simulink model "task3"  (R2024a)
settings: Solver=VariableStepAuto  StartTime=0.0  StopTime=10.0  MaxStep=0.1  RelTol=1e-3
undefined symbols (not defined in the file): A, B, C, D, K, L, x0, x0_hat
settings Model: Creator=sizgr  LastModifiedBy=sizgr

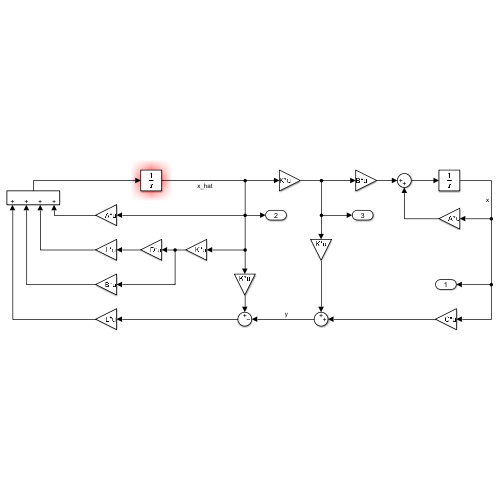
[thumbnail: Simulink's stored preview of the top-level diagram]
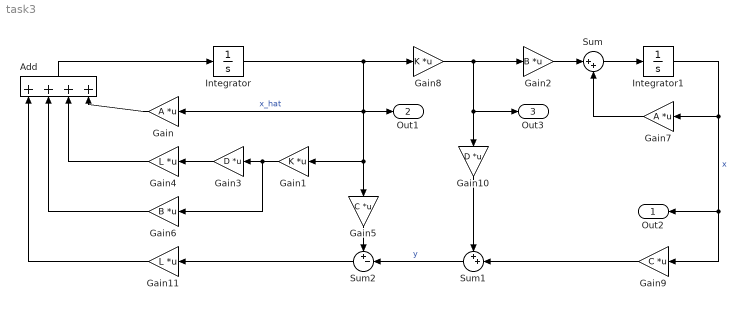
== system task3 ==
  Add : Sum  Inputs=++++
  Gain : Gain  Gain=A  Multiplication=Matrix(K*u)
  Gain1 : Gain  Gain=K  Multiplication=Matrix(K*u)
  Gain10 : Gain  Gain=D  Multiplication=Matrix(K*u)
  Gain11 : Gain  Gain=L  Multiplication=Matrix(K*u)
  Gain2 : Gain  Gain=B  Multiplication=Matrix(K*u)
  Gain3 : Gain  Gain=D  Multiplication=Matrix(K*u)
  Gain4 : Gain  Gain=L  Multiplication=Matrix(K*u)
  Gain5 : Gain  Gain=C  Multiplication=Matrix(K*u)
  Gain6 : Gain  Gain=B  Multiplication=Matrix(K*u)
  Gain7 : Gain  Gain=A  Multiplication=Matrix(K*u)
  Gain8 : Gain  Gain=K  Multiplication=Matrix(K*u)
  Gain9 : Gain  Gain=C  Multiplication=Matrix(K*u)
  Integrator : Integrator  InitialCondition=x0_hat
  Integrator1 : Integrator  InitialCondition=x0
  Sum : Sum  Inputs=|++
  Sum1 : Sum  Inputs=++|
  Sum2 : Sum  Inputs=+-|
  Out2 : Outport
  Out1 : Outport  Port=2
  Out3 : Outport  Port=3
  wires:
  Integrator/1 -> Gain8/1, Out1/1, Gain5/1, Gain1/1, Gain/1  "x_hat"
  Gain3/1 -> Gain4/1
  Gain1/1 -> Gain6/1, Gain3/1
  Integrator1/1 -> Out2/1, Gain9/1, Gain7/1  "x"
  Gain8/1 -> Gain2/1, Out3/1, Gain10/1
  Gain2/1 -> Sum/1
  Sum/1 -> Integrator1/1
  Gain7/1 -> Sum/2
  Gain9/1 -> Sum1/2
  Gain10/1 -> Sum1/1
  Gain5/1 -> Sum2/1
  Sum1/1 -> Sum2/2  "y"
  Sum2/1 -> Gain11/1
  Add/1 -> Integrator/1
  Gain/1 -> Add/4
  Gain4/1 -> Add/3
  Gain6/1 -> Add/2
  Gain11/1 -> Add/1
